simulink model "Cowley_321Project1Sim"  (R2020b)
settings: Solver=VariableStepAuto  StartTime=0.0  StopTime=10.0  RelTol=1e-3
values from neighbouring files (symbols this model uses):
  A = 0.00426    [Cowley_321Lab2.m]    (also in Cowley_321Project2.m = [0 1 0 0 0 0 0 0;-2*ks/m -2*bs/m ks/m bs/m ks/m bs/m ks*(b-a)
  Cd = 0.4    [Cowley_321Lab2.m]
  g = 9.81    [Cowley_321Lab2.m]
  H = 1.85    [Cowley_321Lab2.m]
  m = 0.145    [Cowley_321Lab2.m]    (also in Cowley_321Lab4.m = 2; Cowley_321Project2.m = tand(grade))
  rho = 1.225    [Cowley_321Lab2.m]
  v0x = 40    [Cowley_321Lab2.m]
  v0y = 0    [Cowley_321Lab2.m]
undefined symbols (not defined in the file or in its folder): psi, v0z, vw
settings Model: Creator=mattcowley  LastModifiedBy=mattcowley

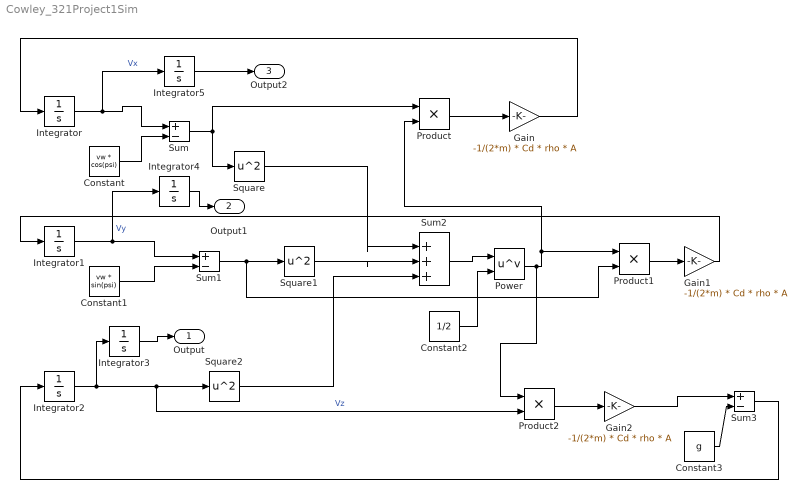
== system Cowley_321Project1Sim ==
  Constant : Constant  Value=vw * cos(psi)
  Constant1 : Constant  Value=vw * sin(psi)
  Constant2 : Constant  Value=1/2
  Constant3 : Constant  Value=g
  Gain : Gain  Gain=-1/(2*m) * Cd * rho * A
  Gain1 : Gain  Gain=-1/(2*m) * Cd * rho * A
  Gain2 : Gain  Gain=-1/(2*m) * Cd * rho * A
  Integrator : Integrator  InitialCondition=v0x
  Integrator1 : Integrator  InitialCondition=v0y
  Integrator2 : Integrator  InitialCondition=v0z
  Integrator3 : Integrator  InitialCondition=H
  Integrator4 : Integrator
  Integrator5 : Integrator
  Power : Math  Operator=pow  SaturateOnIntegerOverflow=on
  Product : Product
  Product1 : Product
  Product2 : Product
  Square : Math  Operator=square  SaturateOnIntegerOverflow=on
  Square1 : Math  Operator=square  SaturateOnIntegerOverflow=on
  Square2 : Math  Operator=square  SaturateOnIntegerOverflow=on
  Sum : Sum  Inputs=+-
  Sum1 : Sum  Inputs=+-
  Sum2 : Sum  Inputs=|+++
  Sum3 : Sum  Inputs=+-
  Output : Outport  SignalName=z
  Output1 : Outport  Port=2  SignalName=y
  Output2 : Outport  Port=3  SignalName=x
  wires:
  Integrator/1 -> Integrator5/1, Sum/1  "Vx"
  Constant/1 -> Sum/2
  Sum/1 -> Product/1, Square/1
  Integrator1/1 -> Integrator4/1, Sum1/1  "Vy"
  Constant1/1 -> Sum1/2
  Sum1/1 -> Product1/2, Square1/1
  Integrator2/1 -> Integrator3/1, Product2/2, Square2/1  "Vz"
  Square2/1 -> Sum2/3
  Square1/1 -> Sum2/2
  Square/1 -> Sum2/1
  Sum2/1 -> Power/1
  Constant2/1 -> Power/2
  Power/1 -> Product2/1, Product1/1, Product/2
  Product/1 -> Gain/1
  Gain/1 -> Integrator/1
  Product1/1 -> Gain1/1
  Gain1/1 -> Integrator1/1
  Product2/1 -> Gain2/1
  Integrator3/1 -> Output/1
  Integrator4/1 -> Output1/1
  Integrator5/1 -> Output2/1
  Constant3/1 -> Sum3/2
  Gain2/1 -> Sum3/1
  Sum3/1 -> Integrator2/1
